simulink model "testModel"  (R2020b)
settings: Solver=VariableStepAuto  StartTime=0.0  StopTime=10.0  RelTol=1e-3
settings Model: Creator=sgaphill  LastModifiedBy=sgaphill
settings SFSimCC: SimCustomHeaderCode="#include \"doubleIt.h\""  SimUserSources=doubleIt.cpp  SimTargetLang=C++

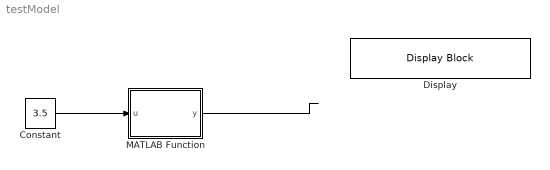
== system testModel ==
  Constant : Constant  Value=3.5
  Display : DisplayBlock  LabelPosition=Hide  Transparency=1
  MATLAB Function : MATLAB Function  TreatAsAtomicUnit=on
  wires:
  Constant/1 -> MATLAB Function/1(u)
  MATLAB Function/1(y) -> ?

== matlab function testModel/MATLAB Function ==
  data: u input; y output
function y = callingDoubleIt(u)

y = 0.0;
y = coder.ceval("doubleIt",u);
